simulink model "imu"  (R2018a)
settings: Solver=FixedStepAuto  StartTime=0.0  StopTime=15  FixedStep=0.01  RelTol=1e-3
values from neighbouring files (symbols this model uses):
  bias = 0.05    [imu_setup.m]
  dt = 0.01    [imu_setup.m]
libraries: simulink x8, simulink_extras x5
settings Model: Creator=Devin  LastModifiedBy=Devin

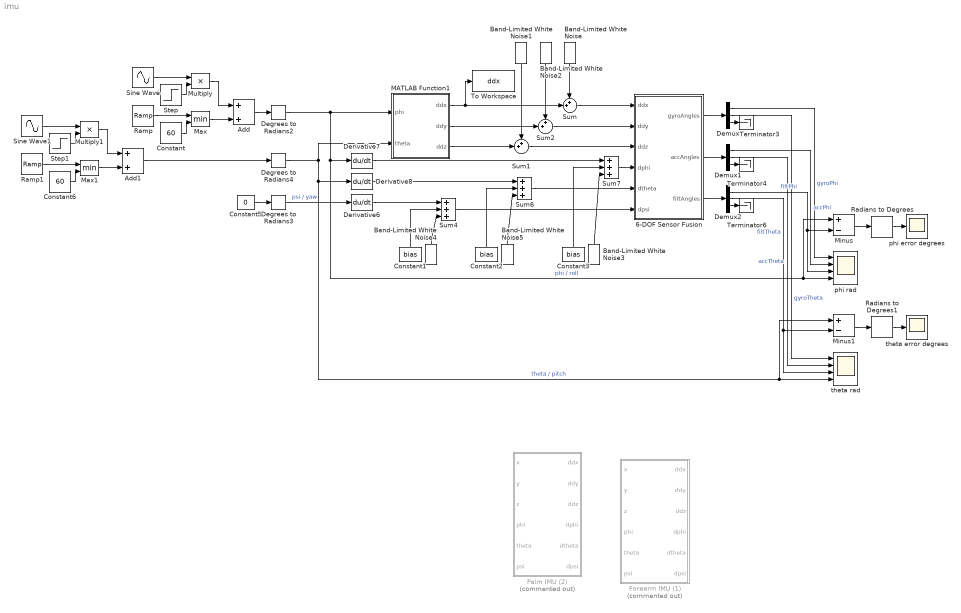
== system imu ==
  6-DOF Sensor Fusion : MATLAB Function  TreatAsAtomicUnit=on
  Add : Sum
  Add1 : Sum
  Band-Limited White Noise : simulink/Sources/Band-Limited White Noise  Cov=0.1  Ts=dt  seed=[23341]
  Band-Limited White Noise1 : simulink/Sources/Band-Limited White Noise  Cov=0.1  Ts=dt  seed=[23311]
  Band-Limited White Noise2 : simulink/Sources/Band-Limited White Noise  Cov=0.1  Ts=dt  seed=[13341]
  Band-Limited White Noise3 : simulink/Sources/Band-Limited White Noise  Cov=0.0001  Ts=dt  seed=[23341]
  Band-Limited White Noise4 : simulink/Sources/Band-Limited White Noise  Cov=0.0001  Ts=dt  seed=[23311]
  Band-Limited White Noise5 : simulink/Sources/Band-Limited White Noise  Cov=0.0001  Ts=dt  seed=[13341]
  Constant : Constant  Value=60
  Constant1 : Constant  Value=bias
  Constant2 : Constant  Value=bias
  Constant3 : Constant  Value=bias
  Constant5 : Constant  Value=0
  Constant6 : Constant  Value=60
  Degrees to Radians2 : simulink_extras/Transformations/Degrees to Radians
  Degrees to Radians3 : simulink_extras/Transformations/Degrees to Radians
  Degrees to Radians4 : simulink_extras/Transformations/Degrees to Radians
  Demux : Demux  Outputs=3
  Demux1 : Demux  Outputs=3
  Demux2 : Demux  Outputs=3
  Derivative6 : Derivative  CoefficientInTFapproximation=0
  Derivative7 : Derivative  CoefficientInTFapproximation=0
  Derivative8 : Derivative  CoefficientInTFapproximation=0
  Forearm IMU (1) : MATLAB Function  Commented=on  TreatAsAtomicUnit=on
  MATLAB Function1 : MATLAB Function  TreatAsAtomicUnit=on
  Max : MinMax  Inputs=2
  Max1 : MinMax  Inputs=2
  Minus : Sum  Inputs=+-
  Minus1 : Sum  Inputs=+-
  Multiply : Product
  Multiply1 : Product
  Palm IMU (2) : MATLAB Function  Commented=on  TreatAsAtomicUnit=on
  Radians to Degrees : simulink_extras/Transformations/Radians to Degrees
  Radians to Degrees1 : simulink_extras/Transformations/Radians to Degrees
  Ramp : simulink/Sources/Ramp  slope=120  start=7  InitialOutput=0
  Ramp1 : simulink/Sources/Ramp  slope=120  start=7  InitialOutput=0
  Sine Wave : Sin  Amplitude=60  Frequency=2  SampleTime=0
  Sine Wave1 : Sin  Amplitude=-30  Frequency=4  SampleTime=0
  Step : Step  Time=5  Before=1  After=0  SampleTime=0
  Step1 : Step  Time=5  Before=1  After=0  SampleTime=0
  Sum : Sum  Inputs=++|
  Sum1 : Sum  Inputs=++|
  Sum2 : Sum  Inputs=++|
  Sum4 : Sum  Inputs=+++
  Sum6 : Sum  Inputs=+++
  Sum7 : Sum  Inputs=+++
  Terminator3 : Terminator
  Terminator4 : Terminator
  Terminator6 : Terminator
  To Workspace : ToWorkspace  VariableName=ddx  SaveFormat=Timeseries  SampleTime=-1
  phi error degrees : Scope
  phi rad : Scope  NumInputPorts=4
  theta error degrees : Scope
  theta rad : Scope  NumInputPorts=4
  wires:
  Degrees to Radians2/1 -> Minus/1, phi rad/4, Derivative7/1, MATLAB Function1/1(phi)  "phi / roll"
  Degrees to Radians4/1 -> MATLAB Function1/2(theta), Minus1/1, theta rad/4, Derivative8/1  "theta / pitch"
  Degrees to Radians3/1 -> Derivative6/1  "psi / yaw"
  MATLAB Function1/1(ddx) -> To Workspace/1, Sum/2
  Sum/1 -> 6-DOF Sensor Fusion/1(ddx)
  Band-Limited White Noise/1 -> Sum/1
  Band-Limited White Noise2/1 -> Sum2/1
  Band-Limited White Noise1/1 -> Sum1/1
  MATLAB Function1/3(ddz) -> Sum1/2
  MATLAB Function1/2(ddy) -> Sum2/2
  Sum2/1 -> 6-DOF Sensor Fusion/2(ddy)
  Sum1/1 -> 6-DOF Sensor Fusion/3(ddz)
  Sum7/1 -> 6-DOF Sensor Fusion/4(dphi)
  Sum6/1 -> 6-DOF Sensor Fusion/5(dtheta)
  Derivative8/1 -> Sum6/1
  Derivative7/1 -> Sum7/1
  Derivative6/1 -> Sum4/1
  Sum4/1 -> 6-DOF Sensor Fusion/6(dpsi)
  Band-Limited White Noise3/1 -> Sum7/3
  Ramp/1 -> Max/1
  Constant/1 -> Max/2
  6-DOF Sensor Fusion/1(gyroAngles) -> Demux/1
  Demux/1 -> phi rad/1  "gyroPhi"
  Demux/2 -> theta rad/1  "gyroTheta"
  Demux/3 -> Terminator3/1
  Add1/1 -> Degrees to Radians4/1
  Constant5/1 -> Degrees to Radians3/1
  Demux1/1 -> phi rad/2  "accPhi"
  6-DOF Sensor Fusion/2(accAngles) -> Demux1/1
  Demux1/2 -> theta rad/2  "accTheta"
  Demux1/3 -> Terminator4/1
  Demux2/1 -> phi rad/3, Minus/2  "filtPhi"
  6-DOF Sensor Fusion/3(filtAngles) -> Demux2/1
  Demux2/2 -> Minus1/2, theta rad/3  "filtTheta"
  Demux2/3 -> Terminator6/1
  Constant1/1 -> Sum4/2
  Band-Limited White Noise4/1 -> Sum4/3
  Constant2/1 -> Sum6/2
  Band-Limited White Noise5/1 -> Sum6/3
  Constant3/1 -> Sum7/2
  Add/1 -> Degrees to Radians2/1
  Max/1 -> Add/2
  Multiply/1 -> Add/1
  Step/1 -> Multiply/2
  Sine Wave/1 -> Multiply/1
  Minus/1 -> Radians to Degrees/1
  Radians to Degrees/1 -> phi error degrees/1
  Multiply1/1 -> Add1/1
  Sine Wave1/1 -> Multiply1/1
  Ramp1/1 -> Max1/1
  Max1/1 -> Add1/2
  Constant6/1 -> Max1/2
  Step1/1 -> Multiply1/2
  Minus1/1 -> Radians to Degrees1/1
  Radians to Degrees1/1 -> theta error degrees/1

== matlab function imu/6-DOF Sensor Fusion ==
  data: ddx input; gyroAngles output; ddy input; ddz input; dphi input; dtheta input; dpsi input; accAngles output; filtAngles output
function [gyroAngles,accAngles,filtAngles] = fuse(ddx,ddy,ddz,dphi,dtheta,dpsi)

%%  Integrate gyro rates to get angles
    % roll = phi, pitch = theta, yaw = psi
    persistent gyroAnglesInternal;
    if isempty(gyroAnglesInternal)
        gyroAnglesInternal = [0; 0; 0];
    end
    
    gyroData = [dphi; dtheta; dpsi];
    
    % sampling time
    dt = 0.01; 
   
    gyroAnglesInternal = gyroAnglesInternal + gyroData * dt;
    gyroAngles = gyroAnglesInternal;
    
%%  Use accelerometer data to get attitude with trig
%   Assumes gravity is primary acceleration being experienced

    accData = [ddx; ddy; ddz];
    g = 9.8;

    % Rot. around x-axis (roll, phi) results in a vector on the y-axis
    accPhi = atan2(accData(2),accData(3));
    % Rot. around y-axis (pitch, theta) results in a vector on the x-axis
    accTheta = -asin(max(min(ddx/g,1),-1));
    
    accAngles = [accPhi; accTheta; 0];
    
%% Combine with complementary filter
    persistent filtAnglesInternal;
    if isempty(filtAnglesInternal)
        filtAnglesInternal = [0;0;0];
    end
    
    filtAnglesInternal = 0.98*(filtAnglesInternal + gyroData * dt) + 0.02*accAngles;
    filtAngles = filtAnglesInternal;

== matlab function imu/Forearm IMU (1) ==
  data: x input; ddx output; y input; z input; phi input; theta input; psi input; ddy output; ddz output; dphi output; dtheta output; dpsi output
function [ddx,ddy,ddz,dphi,dtheta,dpsi] = fcn(x,y,z,phi,theta,psi)

y = u;

== matlab function imu/Palm IMU (2) ==
  data: x input; ddx output; y input; z input; phi input; theta input; psi input; ddy output; ddz output; dphi output; dtheta output; dpsi output
function [ddx,ddy,ddz,dphi,dtheta,dpsi] = fcn(x,y,z,phi,theta,psi)

y = u;

== matlab function imu/MATLAB Function1 ==
  data: phi input; ddx output; theta input; ddy output; ddz output
function [ddx,ddy,ddz]= fcn(phi,theta)
%% turn angles into accelerations, assuming only gravity
g = 9.8;
ddx = -g*sin(theta);
ddy = g*cos(theta)*sin(phi);
ddz = g*cos(theta)*cos(phi);
